simulink model "simThreeLinkFTC"  (R2014b)
settings: Solver=ode45  StartTime=0.0  StopTime=tof  FixedStep=dt  MaxStep=dtmax  RelTol=1e-3
values from neighbouring files (symbols this model uses):
  alpha = 1    [robotArmWith2Links.m]    (also in threeLinkFTC.m; twoLinkFTC.m; twoLinkFTCwAdaptive.m)
  Ar = [0 5; -30 -30]    [robotArmWith2Links.m]    (also in threeLinkFTC.m = [0 1; -5 -5]; twoLinkFTC.m = [0 10; -40 -40]; twoLinkFTCwAdaptive.m = [0 5; -250 -250])
  Arm1 = [0 1; -wn^2 -2*ksi*wn]    [robotArmWith2Links.m]    (also in threeLinkFTC.m; twoLinkFTC.m; twoLinkFTCwAdaptive.m)
  As = zeros(nofstates,nofstates)    [threeLinkFTC.m]    (also in twoLinkFDIbasisComparison.m; twoLinkFTC.m; twoLinkFTCwAdaptive.m)
  Brm1 = [0 wn^2]'    [robotArmWith2Links.m]    (also in threeLinkFTC.m; twoLinkFTC.m; twoLinkFTCwAdaptive.m)
  Dhat0 = zeros(6,1)    [threeLinkFTC.m]    (also in twoLinkFDIbasisComparison.m = zeros(4,1); twoLinkFTC.m = zeros(4,1); twoLinkFTCwAdaptive.m = zeros(4,1))
  Dlimit = 10    [threeLinkFTC.m]    (also in twoLinkFTC.m; twoLinkFTCwAdaptive.m)
  dtFc = 1*dtmax    (= 0.001)    [threeLinkFTC.m]    (also in twoLinkFDIbasisComparison.m; twoLinkFTC.m; twoLinkFTCwAdaptive.m)
  epsilon = 0.5    [robotArmWith2Links.m]    (also in threeLinkFTC.m; twoLinkFTC.m; twoLinkFTCwAdaptive.m)
  epsilontheta = 0.01    [threeLinkFTC.m]    (also in twoLinkFDIbasisComparison.m; twoLinkFTC.m; twoLinkFTCwAdaptive.m)
  faultyArm = 3    [threeLinkFTC.m]    (also in twoLinkFDIbasisComparison.m = 2; twoLinkFTC.m = 2; twoLinkFTCwAdaptive.m = 1)
  FDstart = 0.5    [threeLinkFTC.m]    (also in twoLinkFTC.m; twoLinkFTCwAdaptive.m)
  fmPosition = [0 90 -45]'*pi/180    [threeLinkFTC.m]    (also in twoLinkFTC.m = [90 0]'*pi/180; twoLinkFTCwAdaptive.m = [90 0]'*pi/180)
  g = 9.81    [robotArmWith2Links.m]    (also in threeLinkFTC.m; twoLinkFDIbasisComparison.m; twoLinkFTC.m; twoLinkFTCwAdaptive.m)
  GammaW = 1000    [threeLinkFTC.m]    (also in twoLinkFDIbasisComparison.m; twoLinkFTC.m; twoLinkFTCwAdaptive.m)
  I1 = 8.33e-2    (= 0.0833)    [robotArmWith2Links.m]    (also in threeLinkFTC.m = 0.0833333333333; twoLinkFDIbasisComparison.m = 0.0833333333333; twoLinkFTC.m = 0.0833333333333; twoLinkFTCwAdaptive.m = 0.0833333333333)
  I2 = 8.33e-2    (= 0.0833)    [robotArmWith2Links.m]    (also in threeLinkFTC.m = 0.0833333333333; twoLinkFDIbasisComparison.m = 0.0833333333333; twoLinkFTC.m = 0.0833333333333; twoLinkFTCwAdaptive.m = 0.0833333333333)
  I3 = m3*l3^2*1/12    (= 0.0833333333333)    [threeLinkFTC.m]
  ifault = 2    [threeLinkFTC.m]    (also in twoLinkFDIbasisComparison.m; twoLinkFTC.m; twoLinkFTCwAdaptive.m)
  K1 = 2*wn*ksi    (= 87.9645943005)    [robotArmWith2Links.m]    (also in threeLinkFTC.m = 8.79645943005; twoLinkFTC.m; twoLinkFTCwAdaptive.m = 43.9822971503)
  K2 = wn^2    (= 986.960440109)    [robotArmWith2Links.m]    (also in threeLinkFTC.m = 39.4784176044; twoLinkFTC.m; twoLinkFTCwAdaptive.m)
  Kp = wn^2    (= 157.913670417)    [threeLinkFTC.m]    (also in twoLinkFDIbasisComparison.m = 3947.84176044; twoLinkFTC.m = 3947.84176044; twoLinkFTCwAdaptive.m = 3947.84176044)
  Kv = 2*ksi*wn    (= 17.5929188601)    [threeLinkFTC.m]    (also in twoLinkFDIbasisComparison.m = 125.663706144; twoLinkFTC.m = 125.663706144; twoLinkFTCwAdaptive.m = 125.663706144)
  l1 = 1    [robotArmWith2Links.m]    (also in threeLinkFTC.m; twoLinkFDIbasisComparison.m; twoLinkFTC.m; twoLinkFTCwAdaptive.m)
  l2 = 1    [robotArmWith2Links.m]    (also in threeLinkFTC.m; twoLinkFDIbasisComparison.m; twoLinkFTC.m; twoLinkFTCwAdaptive.m)
  lc1 = l1/2    (= 0.5)    [robotArmWith2Links.m]    (also in threeLinkFTC.m; twoLinkFDIbasisComparison.m; twoLinkFTC.m; twoLinkFTCwAdaptive.m)
  lc2 = l2/2    (= 0.5)    [robotArmWith2Links.m]    (also in threeLinkFTC.m; twoLinkFDIbasisComparison.m; twoLinkFTC.m; twoLinkFTCwAdaptive.m)
  m1 = 1    [robotArmWith2Links.m]    (also in threeLinkFTC.m; twoLinkFDIbasisComparison.m; twoLinkFTC.m; twoLinkFTCwAdaptive.m)
  m2 = 1    [robotArmWith2Links.m]    (also in threeLinkFTC.m; twoLinkFDIbasisComparison.m; twoLinkFTC.m; twoLinkFTCwAdaptive.m)
  m3 = 1    [threeLinkFTC.m]
  nCheby = 4    [threeLinkFTC.m]    (also in twoLinkFDIbasisComparison.m; twoLinkFTC.m; twoLinkFTCwAdaptive.m)
  Ps = lyap(As(4:6,4:6)',Q)    [threeLinkFTC.m]    (also in twoLinkFDIbasisComparison.m = lyap(As(3:4,3:4)',Q); twoLinkFTC.m = lyap(As(3:4,3:4)',Q); twoLinkFTCwAdaptive.m = lyap(As(3:4,3:4)',Q))
  q0 = [80 20]'*pi/180    [robotArmWith2Links.m]    (also in threeLinkFTC.m = [90 0 0]'*pi/180; twoLinkFDIbasisComparison.m = [90 0]'*pi/180; twoLinkFTC.m = [90 0]'*pi/180; twoLinkFTCwAdaptive.m = [90 0]'*pi/180)
  qdot0 = [0 0]'    [robotArmWith2Links.m]    (also in threeLinkFTC.m = [0 0 0]'*pi/180; twoLinkFDIbasisComparison.m = [0 0]'*pi/180; twoLinkFTC.m = [0 0]'*pi/180; twoLinkFTCwAdaptive.m = [0 0]'*pi/180)
  r0 = [0 0]'    [robotArmWith2Links.m]    (also in threeLinkFTC.m; twoLinkFTC.m; twoLinkFTCwAdaptive.m)
  rmax = inf*[50*pi/180 inf]'    [robotArmWith2Links.m]    (also in threeLinkFTC.m; twoLinkFTC.m; twoLinkFTCwAdaptive.m)
  rmin = -rmax    [robotArmWith2Links.m]    (also in threeLinkFTC.m; twoLinkFTC.m; twoLinkFTCwAdaptive.m)
  tfault = 5    [threeLinkFTC.m]    (also in twoLinkFDIbasisComparison.m; twoLinkFTC.m; twoLinkFTCwAdaptive.m = 1)
  W0 = 0    [threeLinkFTC.m]    (also in twoLinkFDIbasisComparison.m; twoLinkFTC.m; twoLinkFTCwAdaptive.m)
  Wbnd = 1000    [threeLinkFTC.m]    (also in twoLinkFDIbasisComparison.m; twoLinkFTC.m; twoLinkFTCwAdaptive.m)
  xhat0 = [q0 ; qdot0]    [threeLinkFTC.m]    (also in twoLinkFDIbasisComparison.m; twoLinkFTC.m; twoLinkFTCwAdaptive.m)
undefined symbols (not defined in the file or in its folder): Intmax, Intmin
libraries: simulink x9, vrlib x3, dspbuff3 x1
(part 2 of 3)

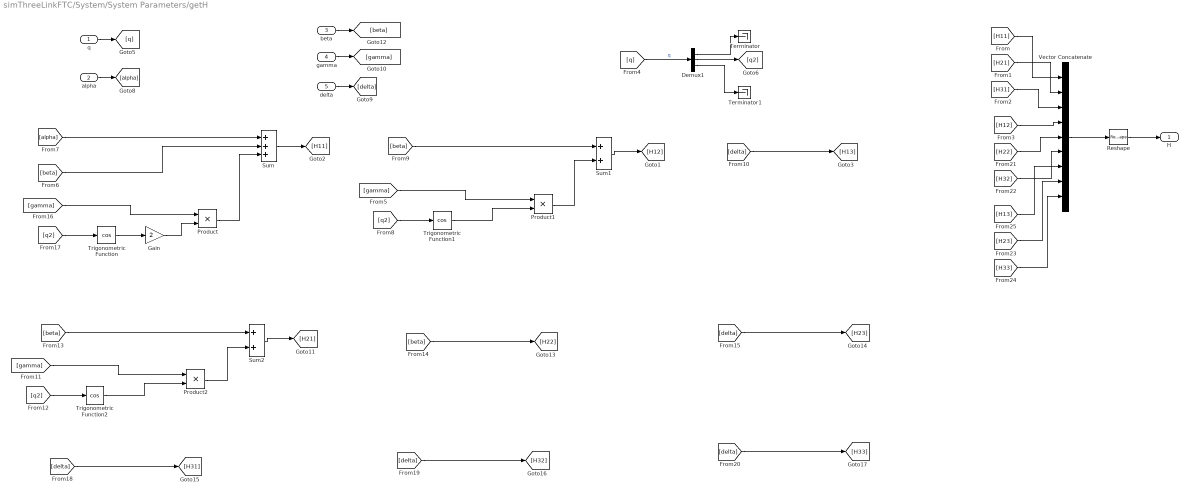
== system simThreeLinkFTC/System/System Parameters/getH ==
  q : Inport
  alpha : Inport  Port=2
  beta : Inport  Port=3
  gamma : Inport  Port=4
  delta : Inport  Port=5
  Demux1 : Demux  Outputs=3
  Gain : Gain  Gain=2
  Product : Product
  Product1 : Product
  Product2 : Product
  Reshape : Reshape  OutputDimensionality=Customize  OutputDimensions=[3,3]
  Sum : Sum  Inputs=+++
  Sum1 : Sum
  Sum2 : Sum
  Terminator : Terminator
  Terminator1 : Terminator
  Trigonometric Function : Trigonometry  Operator=cos
  Trigonometric Function1 : Trigonometry  Operator=cos
  Trigonometric Function2 : Trigonometry  Operator=cos
  Vector Concatenate : Concatenate  NumInputs=9
  H : Outport
  wires:
  Reshape/1 -> H/1
  Sum/1 -> [H11]
  q/1 -> [q]
  [q] -> Demux1/1  "q"
  Demux1/1 -> Terminator/1
  Demux1/3 -> Terminator1/1
  Demux1/2 -> [q2]
  alpha/1 -> [alpha]
  delta/1 -> [delta]
  gamma/1 -> [gamma]
  beta/1 -> [beta]
  [q2] -> Trigonometric Function/1
  Trigonometric Function/1 -> Gain/1
  [gamma] -> Product/1
  Gain/1 -> Product/2
  [alpha] -> Sum/1
  [beta] -> Sum/2
  Product/1 -> Sum/3
  Sum1/1 -> [H12]
  [q2] -> Trigonometric Function1/1
  [gamma] -> Product1/1
  Trigonometric Function1/1 -> Product1/2
  [beta] -> Sum1/1
  Product1/1 -> Sum1/2
  [delta] -> [H13]
  Sum2/1 -> [H21]
  [q2] -> Trigonometric Function2/1
  [gamma] -> Product2/1
  Trigonometric Function2/1 -> Product2/2
  [beta] -> Sum2/1
  Product2/1 -> Sum2/2
  [beta] -> [H22]
  [delta] -> [H23]
  [delta] -> [H31]
  [delta] -> [H32]
  [delta] -> [H33]
  Vector Concatenate/1 -> Reshape/1
  [H12] -> Vector Concatenate/4
  [H22] -> Vector Concatenate/5
  [H31] -> Vector Concatenate/3
  [H32] -> Vector Concatenate/6
  [H21] -> Vector Concatenate/2
  [H11] -> Vector Concatenate/1
  [H13] -> Vector Concatenate/7
  [H23] -> Vector Concatenate/8
  [H33] -> Vector Concatenate/9

== system simThreeLinkFTC/Controller/Disturbance Estimator/getDisturbance/Chebyshev Basis Functions ==
  x : Inport
  tau : Inport  Port=2
  Chebyshev Polynomail Value Calculation : Subsystem  TreatAsAtomicUnit=on
  Demux : Demux  Outputs=6
  Mux : Mux  Inputs=6
  Reshape1 : Reshape  OutputDimensionality=Column vector (2-D)
  Reshape2 : Reshape  OutputDimensionality=Column vector (2-D)
  Terminator1 : Terminator
  Tn : Outport
  wires:
  [Tn] -> Tn/1
  [z] -> Chebyshev Polynomail Value Calculation/1(x)
  Chebyshev Polynomail Value Calculation/1(chebyPol) -> Reshape2/1
  Reshape2/1 -> [Tn]
  tau/1 -> Terminator1/1
  x/1 -> [x]
  Mux/1 -> Reshape1/1
  Reshape1/1 -> [z]
  [x] -> Demux/1
  Demux/1 -> [q1]
  Demux/2 -> [q2]
  Demux/3 -> [q3]
  Demux/4 -> [q1dot]
  Demux/5 -> [q2dot]
  Demux/6 -> [q3dot]
  [q2] -> Mux/2
  [q3] -> Mux/3
  [q1] -> Mux/1
  [q1dot] -> Mux/4
  [q2dot] -> Mux/5
  [q3dot] -> Mux/6

== system simThreeLinkFTC/Controller/Disturbance Estimator/getDisturbance/getDhat ==
  psiz : Inport
  es : Inport  Port=2
  Bus Creator : BusCreator  Inputs=3
  Math Function : Math  Operator=transpose  SaturateOnIntegerOverflow=on
  Math Function1 : Math  Operator=transpose  SaturateOnIntegerOverflow=on
  Math Function2 : Math  Operator=transpose  SaturateOnIntegerOverflow=on
  Reshape : Reshape  OutputDimensionality=Column vector (2-D)
  Selector : Selector  NumberOfDimensions=2  InputPortWidth=3  IndexOptions=Select all,Index vector (dialog)  Indices=[1 3],1  OutputSizes=1,1
  Selector1 : Selector  NumberOfDimensions=2  InputPortWidth=3  IndexOptions=Select all,Index vector (dialog)  Indices=[1 3],2  OutputSizes=1,1
  Selector2 : Selector  NumberOfDimensions=2  InputPortWidth=3  IndexOptions=Select all,Index vector (dialog)  Indices=[1 3],3  OutputSizes=1,1
  Terminator1 : Terminator
  Vector Concatenate : Concatenate  NumInputs=3
  adaptiveGain : Subsystem  TreatAsAtomicUnit=on
  getW1 : Subsystem
  getW2 : Subsystem
  getW3 : Subsystem
  Dhat : Outport
  wires:
  es/1 -> [es]  "es"
  adaptiveGain/1(Wintegrand) -> [Wint]  "Wint"
  [Dhat] -> Dhat/1  "Dhat"
  psiz/1 -> [psiz]  "psiz"
  [es] -> adaptiveGain/2(es)
  [psiz] -> adaptiveGain/1(psi(z))
  [psiz] -> getW1/2(psiz)
  Selector/1 -> getW1/1(Wint)
  Vector Concatenate/1 -> Reshape/1
  [psiz] -> getW2/2(psiz)
  Selector1/1 -> getW2/1(Wint)
  Reshape/1 -> [Dhat]
  Bus Creator/1 -> Terminator1/1  "W"
  getW2/2(WTpsi) -> Vector Concatenate/2
  getW1/2(WTpsi) -> Vector Concatenate/1
  getW1/1(W) -> Math Function/1
  getW2/1(W) -> Math Function1/1
  [Wint] -> Selector2/1, Selector1/1, Selector/1
  Math Function/1 -> Bus Creator/1  "W1"
  Math Function1/1 -> Bus Creator/2  "W2"
  Selector2/1 -> getW3/1(Wint)
  [psiz] -> getW3/2(psiz)
  getW3/1(W) -> Math Function2/1
  Math Function2/1 -> Bus Creator/3
  getW3/2(WTpsi) -> Vector Concatenate/3  "W3"

== system simThreeLinkFTC/Controller/FTC Controller/1st Link Compensator/ ADI Controller ==
  qc : Inport
  q : Inport  Port=2
  qdot : Inport  Port=3
  Comp : Inport  Port=4
  1 : Selector  NumberOfDimensions=2  InputPortWidth=3  IndexOptions=Index vector (dialog),Index vector (dialog)  Indices=1,1  OutputSizes=1,1
  2 : Selector  NumberOfDimensions=2  InputPortWidth=3  IndexOptions=Index vector (dialog),Index vector (dialog)  Indices=1,1  OutputSizes=1,1
  3 : Selector  NumberOfDimensions=2  InputPortWidth=3  IndexOptions=Index vector (dialog),Index vector (dialog)  Indices=2,1  OutputSizes=1,1
  4 : Selector  NumberOfDimensions=2  InputPortWidth=3  IndexOptions=Index vector (dialog),Index vector (dialog)  Indices=2,1  OutputSizes=1,1
  Add : Sum  Inputs=+-+
  Add1 : Sum
  Add2 : Sum
  Constant2 : Constant  Value=2*pi
  Demux : Demux  Outputs=2
  Demux1 : Demux  Outputs=2
  Demux3 : Demux  Outputs=2
  Discrete-Time Integrator : DiscreteIntegrator  IntegratorMethod=Integration: Backward Euler  InitialCondition=r0  InitialConditionSetting=State (most efficient)  SampleTime=-1  LimitOutput=on  UpperSaturationLimit=rmax  LowerSaturationLimit=rmin
  Gain3 : Gain  Gain=[1/epsilon]'
  Gain4 : Gain  Gain=alpha
  Gain8 : Gain  Gain=Ar  Multiplication=Matrix(K*u)
  Math Function : Math  Operator=rem  SaturateOnIntegerOverflow=on
  Memory3 : Memory  X0=r0  InheritSampleTime=on  LinearizeMemory=on  LinearizeAsDelay=on
  Mux1 : Mux  Inputs=2
  Mux2 : Mux  Inputs=2
  Mux3 : Mux  Inputs=2
  Reference model : Subsystem  TreatAsAtomicUnit=on
  Reshape{1..4} (4 alike) : Reshape  OutputDimensionality=Column vector (2-D)
  System model : Subsystem  TreatAsAtomicUnit=on
  Terminator1 : Terminator
  Terminator3 : Terminator
  r : Outport
  wires:
  [Comp] -> Add/3
  Comp/1 -> [Comp]  "Comp"
  [r] -> 4/1
  Reshape4/1 -> r/1  "rp"
  Math Function/1 -> Mux3/2
  Mux3/1 -> Reshape4/1
  4/1 -> Mux3/1
  [r] -> Gain8/1
  1/1 -> Math Function/1
  [r] -> 3/1
  3/1 -> Mux2/2
  Demux1/2 -> Terminator3/1
  [qdot] -> Demux1/1
  Mux2/1 -> Reshape3/1
  Demux1/1 -> Mux2/1
  2/1 -> Add1/2
  [r] -> 2/1
  Demux/2 -> [r2]
  Demux/1 -> [r1]
  Reshape2/1 -> Memory3/1
  Discrete-Time Integrator/1 -> Reshape2/1
  Gain3/1 -> Discrete-Time Integrator/1
  [r] -> 1/1
  Constant2/1 -> Math Function/2
  Memory3/1 -> [r]  "r"
  Add1/1 -> Mux1/2
  [r2] -> Add1/1
  Demux3/2 -> Terminator1/1
  [q] -> Demux3/1
  Reshape1/1 -> System model/1(q)
  Mux1/1 -> Reshape1/1
  Demux3/1 -> Mux1/1
  Reshape3/1 -> System model/2(qdot)
  Gain8/1 -> Add2/2
  System model/1(f1) -> [f1]  "f1"
  Reference model/1(f1r) -> [f1r]  "f1r"
  [r1] -> Reference model/3(r1)  "r1"
  [q] -> Reference model/1(q)
  [qdot] -> Reference model/2(qdot)
  qdot/1 -> [qdot]
  q/1 -> [q]
  Add2/1 -> Gain3/1
  Gain4/1 -> Add2/1
  [f1r] -> Add/2
  [f1] -> Add/1
  Add/1 -> Gain4/1  "r_rhs"
  qc/1 -> Demux/1  "qc"

== system simThreeLinkFTC/Controller/FTC Controller/1st Link Compensator/Partial FBL q2 Controller ==
  qc : Inport
  qcdot : Inport  Port=2
  q : Inport  Port=3
  qdot : Inport  Port=4
  H : Inport  Port=5
  C : Inport  Port=6
  G : Inport  Port=7
  Collocated q2 Controller : Subsystem  TreatAsAtomicUnit=on
  Select 12_1 : Selector  NumberOfDimensions=2  InputPortWidth=3  IndexOptions=Index vector (dialog),Index vector (dialog)  Indices=[2 3],1  OutputSizes=1,1
  Select 12_2 : Selector  NumberOfDimensions=2  InputPortWidth=3  IndexOptions=Index vector (dialog),Index vector (dialog)  Indices=[2 3],1  OutputSizes=1,1
  Torque calculation : Subsystem  TreatAsAtomicUnit=on
  tau : Outport
  v : Outport  Port=2
  wires:
  [qdot] -> Torque calculation/5(qdot)
  Select 12_2/1 -> Collocated q2 Controller/4(qdot)
  [qdot] -> Select 12_2/1
  Select 12_1/1 -> Collocated q2 Controller/3(q)
  qc/1 -> [qc]
  qcdot/1 -> [qcdot]
  [tau] -> tau/1
  [qcdot] -> Collocated q2 Controller/2(rdot)
  [v] -> v/1
  qdot/1 -> [qdot]
  q/1 -> [q]
  [qc] -> Collocated q2 Controller/1(r)
  [G] -> Torque calculation/4(G)
  [C] -> Torque calculation/3(C)
  [H] -> Torque calculation/2(H)
  [v] -> Torque calculation/1(v)
  Torque calculation/1(tau) -> [tau]
  G/1 -> [G]
  H/1 -> [H]
  C/1 -> [C]
  Collocated q2 Controller/1(v) -> [v]  "v"
  [q] -> Select 12_1/1

== system simThreeLinkFTC/Controller/FTC Controller/3rd Link Compensator/ ADI Controller ==
  qc : Inport
  q : Inport  Port=2
  qdot : Inport  Port=3
  Comp : Inport  Port=4
  1 : Selector  NumberOfDimensions=2  InputPortWidth=3  IndexOptions=Index vector (dialog),Index vector (dialog)  Indices=1,1  OutputSizes=1,1
  3 : Selector  InputPortWidth=2  Indices=2
  4 : Selector  NumberOfDimensions=2  InputPortWidth=3  IndexOptions=Index vector (dialog),Index vector (dialog)  Indices=2,1  OutputSizes=1,1
  5 : Selector  InputPortWidth=2
  Add : Sum  Inputs=+-+
  Add1 : Sum
  Add2 : Sum
  Constant2 : Constant  Value=2*pi
  Discrete-Time Integrator : DiscreteIntegrator  IntegratorMethod=Integration: Backward Euler  InitialCondition=r0  InitialConditionSetting=State (most efficient)  SampleTime=-1  LimitOutput=on  UpperSaturationLimit=rmax  LowerSaturationLimit=rmin
  Gain3 : Gain  Gain=[1/epsilon]'
  Gain4 : Gain  Gain=alpha
  Gain8 : Gain  Gain=Ar  Multiplication=Matrix(K*u)
  Math Function : Math  Operator=rem  SaturateOnIntegerOverflow=on
  Memory3 : Memory  X0=r0  InheritSampleTime=on  LinearizeMemory=on  LinearizeAsDelay=on
  Mux1 : Mux  Inputs=3
  Mux2 : Mux  Inputs=3
  Mux3 : Mux  Inputs=2
  Reference model : Subsystem  TreatAsAtomicUnit=on
  Reshape{1..4} (4 alike) : Reshape  OutputDimensionality=Column vector (2-D)
  Selec t 1 : Selector  InputPortWidth=3
  Selec t 2 : Selector  InputPortWidth=3
  Selec t 3 : Selector  NumberOfDimensions=2  InputPortWidth=3  IndexOptions=Index vector (dialog),Index vector (dialog)  Indices=3,1  OutputSizes=1,1
  Selec t 4 : Selector  InputPortWidth=3  Indices=3
  Selec t 5 : Selector  InputPortWidth=3  Indices=3
  Selec t 6 : Selector  NumberOfDimensions=2  InputPortWidth=3  IndexOptions=Index vector (dialog),Index vector (dialog)  Indices=[1 2],1  OutputSizes=1,1
  System model : Subsystem  TreatAsAtomicUnit=on
  r : Outport
  wires:
  Add/1 -> Gain4/1  "r_rhs"
  [f1] -> Add/1
  [f1r] -> Add/2
  Gain4/1 -> Add2/1
  Add2/1 -> Gain3/1
  q/1 -> [q]
  qdot/1 -> [qdot]
  [qdot] -> Reference model/2(qdot)
  [q] -> Reference model/1(q)
  [r1] -> Reference model/3(r1)  "r1"
  Reference model/1(f1r) -> [f1r]  "f1r"
  System model/1(f1) -> [f1]  "f1"
  Gain8/1 -> Add2/2
  Reshape3/1 -> System model/2(qdot)
  Mux1/1 -> Reshape1/1
  Reshape1/1 -> System model/1(q)
  [r2] -> Add1/1
  Add1/1 -> Mux1/2
  Memory3/1 -> [r]  "r"
  Constant2/1 -> Math Function/2
  [r] -> 1/1
  Gain3/1 -> Discrete-Time Integrator/1
  Discrete-Time Integrator/1 -> Reshape2/1
  Reshape2/1 -> Memory3/1
  [r] -> 5/1
  5/1 -> Add1/2
  Mux2/1 -> Reshape3/1
  3/1 -> Mux2/2
  [r] -> 3/1
  1/1 -> Math Function/1
  [r] -> Gain8/1
  Mux3/1 -> Reshape4/1
  Reshape4/1 -> r/1  "rp"
  [r] -> 4/1
  Comp/1 -> [Comp]  "Comp"
  [Comp] -> Add/3
  qc/1 -> Selec t 3/1, Selec t 6/1  "qc"
  Selec t 3/1 -> [r1]
  [q] -> Selec t 1/1
  Selec t 1/1 -> Mux1/1
  [qdot] -> Selec t 2/1
  Selec t 2/1 -> Mux2/1
  [q] -> Selec t 4/1
  Selec t 4/1 -> Mux1/3
  [qdot] -> Selec t 5/1
  Selec t 5/1 -> Mux2/3
  Selec t 6/1 -> [r2]
  Math Function/1 -> Mux3/1
  4/1 -> Mux3/2

== system simThreeLinkFTC/Controller/FTC Controller/3rd Link Compensator/Partial FBL q2 Controller ==
  qc : Inport
  qcdot : Inport  Port=2
  q : Inport  Port=3
  qdot : Inport  Port=4
  H : Inport  Port=5
  C : Inport  Port=6
  G : Inport  Port=7
  Collocated q2 Controller : Subsystem  TreatAsAtomicUnit=on
  Select 12_1 : Selector  NumberOfDimensions=2  InputPortWidth=3  IndexOptions=Index vector (dialog),Index vector (dialog)  Indices=[1 2],1  OutputSizes=1,1
  Select 12_2 : Selector  NumberOfDimensions=2  InputPortWidth=3  IndexOptions=Index vector (dialog),Index vector (dialog)  Indices=[1 2],1  OutputSizes=1,1
  Torque calculation : Subsystem  TreatAsAtomicUnit=on
  tau : Outport
  v : Outport  Port=2
  wires:
  [q] -> Select 12_1/1
  Collocated q2 Controller/1(v) -> [v]  "v"
  C/1 -> [C]
  H/1 -> [H]
  G/1 -> [G]
  Torque calculation/1(tau) -> [tau]
  [v] -> Torque calculation/1(v)
  [H] -> Torque calculation/2(H)
  [C] -> Torque calculation/3(C)
  [G] -> Torque calculation/4(G)
  [qc] -> Collocated q2 Controller/1(r)
  q/1 -> [q]
  qdot/1 -> [qdot]
  [v] -> v/1
  [qcdot] -> Collocated q2 Controller/2(rdot)
  [tau] -> tau/1
  qcdot/1 -> [qcdot]
  qc/1 -> [qc]
  Select 12_1/1 -> Collocated q2 Controller/3(q)
  [qdot] -> Select 12_2/1
  Select 12_2/1 -> Collocated q2 Controller/4(qdot)
  [qdot] -> Torque calculation/5(qdot)

== system simThreeLinkFTC/Controller/Disturbance Estimator/getDisturbance/Chebyshev Basis Functions/Chebyshev Polynomail Value Calculation ==
  x : Inport
  Delay Line : dspbuff3/Delay Line  siz=nCheby  ic=zeros(nCheby,1)  directfeed=on  enable_output=off  hold_output=off  TreatMby1Signals=M channels (this choice will be removed - see release notes)
  For Iterator : ForIterator  IterationLimit=nCheby
  Frame Conversion : FrameConversion  OutFrame=Sample-based
  If : If  IfExpression=u1 > 2
  If Action Subsystem : Subsystem  TreatAsAtomicUnit=on
  If Action Subsystem1 : Subsystem  TreatAsAtomicUnit=on
  Memory : Memory  InheritSampleTime=on  LinearizeMemory=on  LinearizeAsDelay=on
  Merge : Merge
  Reshape : Reshape  OutputDimensionality=Column vector (2-D)
  chebyPol : Outport
  wires:
  For Iterator/1 -> [N]
  x/1 -> [x]
  [N] -> If/1
  If/1 -> If Action Subsystem/Action
  If/2 -> If Action Subsystem1/Action
  [N] -> If Action Subsystem1/2(N)
  [x] -> If Action Subsystem1/1(x)
  [x] -> If Action Subsystem/1(x)
  If Action Subsystem/1(polyval) -> Merge/1
  If Action Subsystem1/1(polval) -> Merge/2
  Merge/1 -> [polyval]
  [polyval] -> Delay Line/1
  Delay Line/1 -> Frame Conversion/1
  Reshape/1 -> [polyvals]
  [polyvals] -> Memory/1
  [polyvals] -> chebyPol/1  "chebyPol"
  Frame Conversion/1 -> Reshape/1
  Memory/1 -> If Action Subsystem/2(polyvals)

== system simThreeLinkFTC/Controller/Disturbance Estimator/getDisturbance/getDhat/adaptiveGain ==
  psi(z) : Inport
  es : Inport  Port=2
  Gain1 : Gain  Gain=-1
  Math Function : Math  Operator=transpose  SaturateOnIntegerOverflow=on
  P : Constant  Value=Ps  VectorParams1D=off
  Product1 : Product  Multiplication=Matrix(*)  RndMeth=Zero
  Product3 : Product  Multiplication=Matrix(*)  RndMeth=Zero
  Wintegrand : Outport
  wires:
  Product1/1 -> Product3/2
  psi(z)/1 -> Product3/1
  Gain1/1 -> Wintegrand/1
  es/1 -> Math Function/1
  Math Function/1 -> Product1/1
  P/1 -> Product1/2
  Product3/1 -> Gain1/1

== system simThreeLinkFTC/Controller/Disturbance Estimator/getDisturbance/getDhat/getW1 ==
  Wint : Inport
  psiz : Inport  Port=2
  Constant : Constant  Value=Wbnd  VectorParams1D=off
  Constant1 : Constant  Value=epsilontheta
  Discrete-Time Integrator : DiscreteIntegrator  IntegratorMethod=Integration: Trapezoidal  InitialCondition=W0  SampleTime=-1  LimitOutput=on  UpperSaturationLimit=Wbnd  LowerSaturationLimit=-Wbnd
  Gain : Gain  Gain=GammaW
  Math Function : Math  Operator=transpose  SaturateOnIntegerOverflow=on
  Memory4 : Memory  X0=W0  InheritSampleTime=on  LinearizeMemory=on  LinearizeAsDelay=on
  Product : Product  Multiplication=Matrix(*)  RndMeth=Zero
  Projection : Subsystem  TreatAsAtomicUnit=on
  W : Outport
  WTpsi : Outport  Port=2
  wires:
  [WTpsi] -> WTpsi/1
  [Wint] -> Projection/2(y)
  Math Function/1 -> Product/1
  [psiz] -> Product/2
  Discrete-Time Integrator/1 -> Math Function/1, [W], Memory4/1
  Gain/1 -> Discrete-Time Integrator/1
  Projection/1(Proj) -> Gain/1  "WintProj"
  Memory4/1 -> Projection/1(theta)
  Constant/1 -> Projection/3(Thetamax)
  Constant1/1 -> Projection/4(epsilontheta)
  [W] -> W/1
  Wint/1 -> [Wint]
  psiz/1 -> [psiz]
  Product/1 -> [WTpsi]  "WTpsi"

== system simThreeLinkFTC/Controller/Disturbance Estimator/getDisturbance/getDhat/getW2 ==
  Wint : Inport
  psiz : Inport  Port=2
  Constant : Constant  Value=Wbnd  VectorParams1D=off
  Constant1 : Constant  Value=epsilontheta
  Discrete-Time Integrator : DiscreteIntegrator  IntegratorMethod=Integration: Trapezoidal  InitialCondition=W0  SampleTime=-1  LimitOutput=on  UpperSaturationLimit=Wbnd  LowerSaturationLimit=-Wbnd
  Gain : Gain  Gain=GammaW
  Math Function : Math  Operator=transpose  SaturateOnIntegerOverflow=on
  Memory4 : Memory  X0=W0  InheritSampleTime=on  LinearizeMemory=on  LinearizeAsDelay=on
  Product : Product  Multiplication=Matrix(*)  RndMeth=Zero
  Projection : Subsystem  TreatAsAtomicUnit=on
  W : Outport
  WTpsi : Outport  Port=2
  wires:
  Product/1 -> [WTpsi]  "WTpsi"
  psiz/1 -> [psiz]
  Wint/1 -> [Wint]
  [W] -> W/1
  Constant1/1 -> Projection/4(epsilontheta)
  Constant/1 -> Projection/3(Thetamax)
  Memory4/1 -> Projection/1(theta)
  Projection/1(Proj) -> Gain/1  "WintProj"
  Gain/1 -> Discrete-Time Integrator/1
  Discrete-Time Integrator/1 -> Memory4/1, [W], Math Function/1
  [psiz] -> Product/2
  Math Function/1 -> Product/1
  [Wint] -> Projection/2(y)
  [WTpsi] -> WTpsi/1

== system simThreeLinkFTC/Controller/Disturbance Estimator/getDisturbance/getDhat/getW3 ==
  Wint : Inport
  psiz : Inport  Port=2
  Constant : Constant  Value=Wbnd  VectorParams1D=off
  Constant1 : Constant  Value=epsilontheta
  Discrete-Time Integrator : DiscreteIntegrator  IntegratorMethod=Integration: Trapezoidal  InitialCondition=W0  SampleTime=-1  LimitOutput=on  UpperSaturationLimit=Wbnd  LowerSaturationLimit=-Wbnd
  Gain : Gain  Gain=GammaW
  Math Function : Math  Operator=transpose  SaturateOnIntegerOverflow=on
  Memory4 : Memory  X0=W0  InheritSampleTime=on  LinearizeMemory=on  LinearizeAsDelay=on
  Product : Product  Multiplication=Matrix(*)  RndMeth=Zero
  Projection : Subsystem  TreatAsAtomicUnit=on
  W : Outport
  WTpsi : Outport  Port=2
  wires:
  [WTpsi] -> WTpsi/1
  [Wint] -> Projection/2(y)
  Math Function/1 -> Product/1
  [psiz] -> Product/2
  Discrete-Time Integrator/1 -> Math Function/1, [W], Memory4/1
  Gain/1 -> Discrete-Time Integrator/1
  Projection/1(Proj) -> Gain/1  "WintProj"
  Memory4/1 -> Projection/1(theta)
  Constant/1 -> Projection/3(Thetamax)
  Constant1/1 -> Projection/4(epsilontheta)
  [W] -> W/1
  Wint/1 -> [Wint]
  psiz/1 -> [psiz]
  Product/1 -> [WTpsi]  "WTpsi"

== system simThreeLinkFTC/Controller/FTC Controller/1st Link Compensator/ ADI Controller/Reference model ==
  q : Inport
  qdot : Inport  Port=2
  r1 : Inport  Port=3
  Add : Sum
  Constant : Constant  Value=Arm1  VectorParams1D=off
  Constant1 : Constant  Value=Brm1  VectorParams1D=off
  Demux2 : Demux  Outputs=2
  Demux3 : Demux  Outputs=2
  Mux : Mux  Inputs=2
  Product1 : Product  Multiplication=Matrix(*)
  Product3 : Product  Multiplication=Matrix(*)
  Reshape : Reshape  OutputDimensionality=Column vector (2-D)
  Terminator4 : Terminator
  Terminator5 : Terminator
  f1r : Outport
  wires:
  Add/1 -> [f1r]
  Product1/1 -> Add/2
  Product3/1 -> Add/1
  [r1] -> Product1/2
  Constant1/1 -> Product1/1
  Reshape/1 -> Product3/2
  Mux/1 -> Reshape/1
  [q1] -> Mux/1
  [q1dot] -> Mux/2
  [q2] -> Terminator5/1
  [q2dot] -> Terminator4/1
  [f1r] -> f1r/1
  Constant/1 -> Product3/1
  r1/1 -> [r1]
  Demux2/1 -> [q1]
  Demux2/2 -> [q2]
  Demux3/1 -> [q1dot]
  Demux3/2 -> [q2dot]
  q/1 -> Demux2/1
  qdot/1 -> Demux3/1

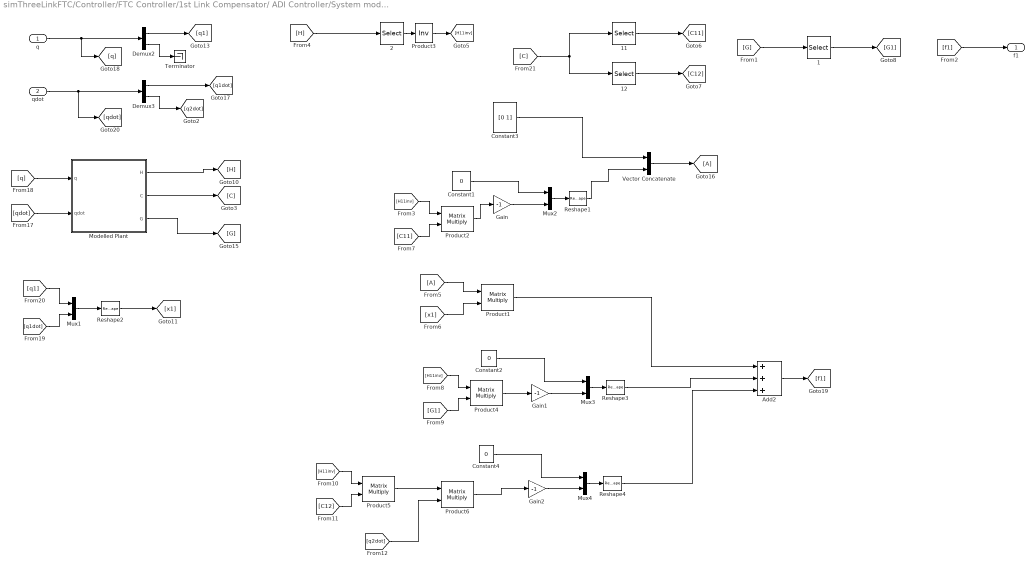
== system simThreeLinkFTC/Controller/FTC Controller/1st Link Compensator/ ADI Controller/System model ==
  q : Inport
  qdot : Inport  Port=2
  1 : Selector  NumberOfDimensions=2  InputPortWidth=3  IndexOptions=Index vector (dialog),Index vector (dialog)  Indices=1,1  OutputSizes=1,1
  11 : Selector  NumberOfDimensions=2  InputPortWidth=3  IndexOptions=Index vector (dialog),Index vector (dialog)  Indices=1,1  OutputSizes=1,1
  12 : Selector  NumberOfDimensions=2  InputPortWidth=3  IndexOptions=Index vector (dialog),Index vector (dialog)  Indices=1,2  OutputSizes=1,1
  2 : Selector  NumberOfDimensions=2  InputPortWidth=3  IndexOptions=Index vector (dialog),Index vector (dialog)  Indices=1,1  OutputSizes=1,1
  Add2 : Sum  Inputs=+++
  Constant1 : Constant  Value=0  VectorParams1D=off
  Constant2 : Constant  Value=0  VectorParams1D=off
  Constant3 : Constant  Value=[0 1]  VectorParams1D=off
  Constant4 : Constant  Value=0  VectorParams1D=off
  Demux2 : Demux  Outputs=2
  Demux3 : Demux  Outputs=2
  Gain : Gain  Gain=-1
  Gain1 : Gain  Gain=-1
  Gain2 : Gain  Gain=-1
  Modelled Plant : Subsystem  TreatAsAtomicUnit=on
  Mux{1..4} (4 alike) : Mux  Inputs=2
  Product{1..2,4..6} (5 alike) : Product  Multiplication=Matrix(*)  RndMeth=Zero
  Product3 : Product  Inputs=/  Multiplication=Matrix(*)  RndMeth=Zero
  Reshape1 : Reshape  OutputDimensionality=Row vector (2-D)
  Reshape2 : Reshape  OutputDimensionality=Column vector (2-D)
  Reshape3 : Reshape  OutputDimensionality=Column vector (2-D)
  Reshape4 : Reshape  OutputDimensionality=Column vector (2-D)
  Terminator : Terminator
  Vector Concatenate : Concatenate  Mode=Multidimensional array
  f1 : Outport
  wires:
  Reshape4/1 -> Add2/3
  Reshape3/1 -> Add2/2
  Product6/1 -> Gain2/1
  [q2dot] -> Product6/2
  Product5/1 -> Product6/1
  Gain2/1 -> Mux4/2
  Mux4/1 -> Reshape4/1
  Constant4/1 -> Mux4/1
  [C12] -> Product5/2
  [H11inv] -> Product5/1
  Gain1/1 -> Mux3/2
  Mux3/1 -> Reshape3/1
  Constant2/1 -> Mux3/1
  Product4/1 -> Gain1/1
  Gain/1 -> Mux2/2
  [G1] -> Product4/2
  [H11inv] -> Product4/1
  [x1] -> Product1/2
  [A] -> Product1/1
  Vector Concatenate/1 -> [A]
  Reshape1/1 -> Vector Concatenate/2
  Constant3/1 -> Vector Concatenate/1
  Mux2/1 -> Reshape1/1
  Constant1/1 -> Mux2/1
  Product2/1 -> Gain/1
  Reshape2/1 -> [x1]
  Mux1/1 -> Reshape2/1
  [q1] -> Mux1/1
  [q1dot] -> Mux1/2
  [q] -> Modelled Plant/1(q)
  [qdot] -> Modelled Plant/2(qdot)
  Modelled Plant/3(G) -> [G]
  Modelled Plant/2(C) -> [C]
  Modelled Plant/1(H) -> [H]
  [C11] -> Product2/2
  [H11inv] -> Product2/1
  Add2/1 -> [f1]
  Product1/1 -> Add2/1
  Product3/1 -> [H11inv]
  2/1 -> Product3/1
  [H] -> 2/1
  Demux2/1 -> [q1]
  Demux2/2 -> Terminator/1
  Demux3/1 -> [q1dot]
  Demux3/2 -> [q2dot]
  q/1 -> Demux2/1, [q]
  qdot/1 -> Demux3/1, [qdot]
  1/1 -> [G1]
  [G] -> 1/1
  12/1 -> [C12]
  11/1 -> [C11]
  [C] -> 11/1, 12/1
  [f1] -> f1/1

== system simThreeLinkFTC/Controller/FTC Controller/1st Link Compensator/Partial FBL q2 Controller/Collocated q2 Controller ==
  r : Inport
  rdot : Inport  Port=2
  q : Inport  Port=3
  qdot : Inport  Port=4
  Add3 : Sum
  Gain2 : Gain  Gain=-K1
  Gain3 : Gain  Gain=-K2
  sum1 : Sum  Inputs=+-
  sum2 : Sum  Inputs=+-
  v : Outport
  wires:
  rdot/1 -> [rdot]  "rdot"
  sum2/1 -> [edot]  "edot"
  [rdot] -> sum2/2
  [qdot] -> sum2/1
  [v] -> v/1  "v"
  r/1 -> [r]  "r"
  sum1/1 -> [e]  "e"
  [r] -> sum1/2
  [q] -> sum1/1
  q/1 -> [q]  "q"
  qdot/1 -> [qdot]  "qdot"
  [edot] -> Gain2/1
  [e] -> Gain3/1
  Gain2/1 -> Add3/1
  Gain3/1 -> Add3/2
  Add3/1 -> [v]

== system simThreeLinkFTC/Controller/FTC Controller/1st Link Compensator/Partial FBL q2 Controller/Torque calculation ==
  v : Inport
  H : Inport  Port=2
  C : Inport  Port=3
  G : Inport  Port=4
  qdot : Inport  Port=5
  1 : Selector  NumberOfDimensions=2  InputPortWidth=3  IndexOptions=Index vector (dialog),Index vector (dialog)  Indices=[1],1  OutputSizes=1,1
  11 : Selector  NumberOfDimensions=2  InputPortWidth=3  IndexOptions=Index vector (dialog),Index vector (dialog)  Indices=1,1  OutputSizes=1,1
  12-13 : Selector  NumberOfDimensions=2  InputPortWidth=3  IndexOptions=Index vector (dialog),Index vector (dialog)  Indices=1,[2 3]  OutputSizes=1,1
  2-3 : Selector  NumberOfDimensions=2  InputPortWidth=3  IndexOptions=Index vector (dialog),Index vector (dialog)  Indices=[2 3],1  OutputSizes=1,1
  21-31 : Selector  NumberOfDimensions=2  InputPortWidth=3  IndexOptions=Index vector (dialog),Index vector (dialog)  Indices=[2 3],1  OutputSizes=1,1
  22-33 : Selector  NumberOfDimensions=2  InputPortWidth=3  IndexOptions=Index vector (dialog),Index vector (dialog)  Indices=[2 3],[2 3]  OutputSizes=1,1
  Product : Product  Inputs=/  Multiplication=Matrix(*)  RndMeth=Zero
  Product{1..4,6..7} (6 alike) : Product  Multiplication=Matrix(*)  RndMeth=Zero
  Product5 : Product  Inputs=/  Multiplication=Matrix(*)  RndMeth=Zero
  Sum of Elements1 : Sum  Inputs=+-+
  Sum of Elements2 : Sum
  Sum of Elements3 : Sum  Inputs=+-
  tau : Outport
  wires:
  [qdotp] -> [qdot]
  qdot/1 -> [qdotp]
  2-3/1 -> [Phi2]
  1/1 -> [Phi1]
  22-33/1 -> [H22]
  21-31/1 -> [H21]
  12-13/1 -> [H12]
  11/1 -> [H11]
  Sum of Elements2/1 -> 2-3/1, 1/1
  [G] -> Sum of Elements2/2
  Product2/1 -> Sum of Elements2/1
  [qdot] -> Product2/2
  [C] -> Product2/1
  [Hp] -> 22-33/1, 21-31/1, 12-13/1, 11/1
  G/1 -> [Gp]
  H/1 -> [Hp]
  C/1 -> [Cp]
  Product3/1 -> Sum of Elements1/3
  Product4/1 -> Sum of Elements1/2
  [Phi2] -> Sum of Elements1/1
  [Phi1] -> Product4/2
  Sum of Elements3/1 -> [Hbar]
  Product7/1 -> Sum of Elements3/2
  [H22] -> Sum of Elements3/1
  [H12] -> Product7/2
  Product6/1 -> Product7/1
  Product5/1 -> Product6/2
  [H21] -> Product6/1
  [H11] -> Product5/1
  Sum of Elements1/1 -> [tau]
  [v] -> Product3/2
  [Hbar] -> Product3/1
  Product1/1 -> Product4/1
  Product/1 -> Product1/2
  [H21] -> Product1/1
  [H11] -> Product/1
  v/1 -> [v]
  [tau] -> tau/1
  [Gp] -> [G]
  [Cp] -> [C]

== system simThreeLinkFTC/Controller/FTC Controller/3rd Link Compensator/ ADI Controller/Reference model ==
  q : Inport
  qdot : Inport  Port=2
  r1 : Inport  Port=3
  Add : Sum
  Constant : Constant  Value=Arm1  VectorParams1D=off
  Constant1 : Constant  Value=Brm1  VectorParams1D=off
  Mux : Mux  Inputs=2
  Product1 : Product  Multiplication=Matrix(*)
  Product3 : Product  Multiplication=Matrix(*)
  Reshape : Reshape  OutputDimensionality=Column vector (2-D)
  Selec t 1 : Selector  NumberOfDimensions=2  InputPortWidth=3  IndexOptions=Index vector (dialog),Index vector (dialog)  Indices=3,1  OutputSizes=1,1
  Selec t 3 : Selector  NumberOfDimensions=2  InputPortWidth=3  IndexOptions=Index vector (dialog),Index vector (dialog)  Indices=3,1  OutputSizes=1,1
  f1r : Outport
  wires:
  q/1 -> Selec t 3/1
  r1/1 -> [r1]
  Constant/1 -> Product3/1
  [f1r] -> f1r/1
  [q1dot] -> Mux/2
  [q1] -> Mux/1
  Mux/1 -> Reshape/1
  Reshape/1 -> Product3/2
  Constant1/1 -> Product1/1
  [r1] -> Product1/2
  Product3/1 -> Add/1
  Product1/1 -> Add/2
  Add/1 -> [f1r]
  Selec t 3/1 -> [q1]
  qdot/1 -> Selec t 1/1
  Selec t 1/1 -> [q1dot]

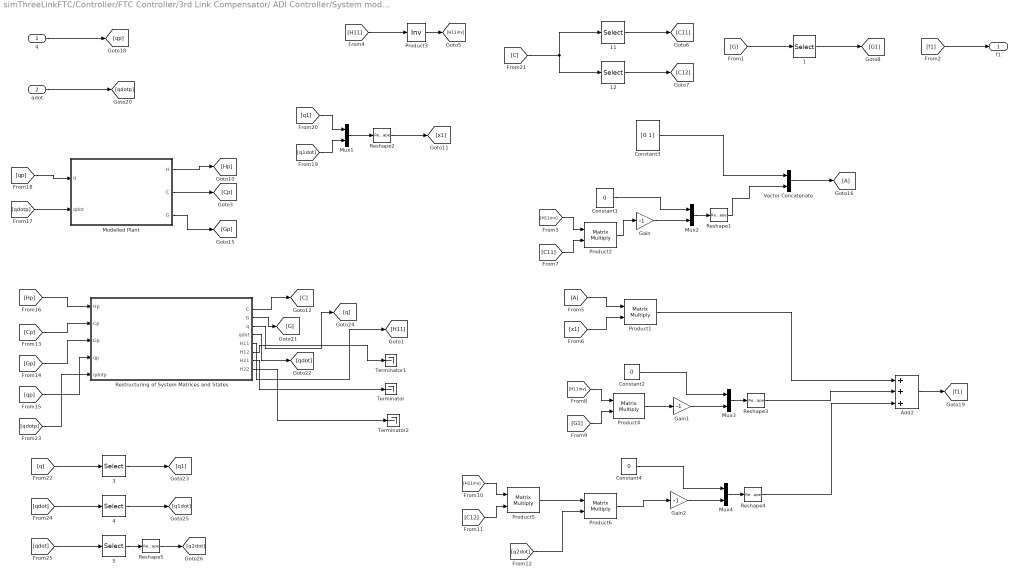
== system simThreeLinkFTC/Controller/FTC Controller/3rd Link Compensator/ ADI Controller/System model ==
  q : Inport
  qdot : Inport  Port=2
  1 : Selector  NumberOfDimensions=2  InputPortWidth=3  IndexOptions=Index vector (dialog),Index vector (dialog)  Indices=1,1  OutputSizes=1,1
  11 : Selector  NumberOfDimensions=2  InputPortWidth=3  IndexOptions=Index vector (dialog),Index vector (dialog)  Indices=1,1  OutputSizes=1,1
  12 : Selector  NumberOfDimensions=2  InputPortWidth=3  IndexOptions=Index vector (dialog),Index vector (dialog)  Indices=1,[2 3]  OutputSizes=1,1
  3 : Selector  InputPortWidth=3
  4 : Selector  InputPortWidth=3
  5 : Selector  InputPortWidth=3  Indices=[2 3]
  Add2 : Sum  Inputs=+++
  Constant1 : Constant  Value=0  VectorParams1D=off
  Constant2 : Constant  Value=0  VectorParams1D=off
  Constant3 : Constant  Value=[0 1]  VectorParams1D=off
  Constant4 : Constant  Value=0  VectorParams1D=off
  Gain : Gain  Gain=-1
  Gain1 : Gain  Gain=-1
  Gain2 : Gain  Gain=-1
  Modelled Plant : Subsystem
  Mux{1..4} (4 alike) : Mux  Inputs=2
  Product{1..2,4..6} (5 alike) : Product  Multiplication=Matrix(*)  RndMeth=Zero
  Product3 : Product  Inputs=/  Multiplication=Matrix(*)  RndMeth=Zero
  Reshape1 : Reshape  OutputDimensionality=Row vector (2-D)
  Reshape{2..5} (4 alike) : Reshape  OutputDimensionality=Column vector (2-D)
  Restructuring of System Matrices and States : Subsystem
  Terminator : Terminator
  Terminator1 : Terminator
  Terminator2 : Terminator
  Vector Concatenate : Concatenate  Mode=Multidimensional array
  f1 : Outport
  wires:
  [f1] -> f1/1
  [C] -> 12/1, 11/1
  11/1 -> [C11]
  12/1 -> [C12]
  [G] -> 1/1
  1/1 -> [G1]
  qdot/1 -> [qdotp]
  [H11] -> Product3/1
  Product3/1 -> [H11inv]
  Product1/1 -> Add2/1
  Add2/1 -> [f1]
  [H11inv] -> Product2/1
  [C11] -> Product2/2
  Modelled Plant/1(H) -> [Hp]
  Modelled Plant/2(C) -> [Cp]
  Modelled Plant/3(G) -> [Gp]
  [qdotp] -> Modelled Plant/2(qdot)
  [q1dot] -> Mux1/2
  [q1] -> Mux1/1
  Mux1/1 -> Reshape2/1
  Reshape2/1 -> [x1]
  Product2/1 -> Gain/1
  Constant1/1 -> Mux2/1
  Mux2/1 -> Reshape1/1
  Constant3/1 -> Vector Concatenate/1
  Reshape1/1 -> Vector Concatenate/2
  Vector Concatenate/1 -> [A]
  [A] -> Product1/1
  [x1] -> Product1/2
  [H11inv] -> Product4/1
  [G1] -> Product4/2
  Gain/1 -> Mux2/2
  Product4/1 -> Gain1/1
  Constant2/1 -> Mux3/1
  Mux3/1 -> Reshape3/1
  Gain1/1 -> Mux3/2
  [H11inv] -> Product5/1
  [C12] -> Product5/2
  Constant4/1 -> Mux4/1
  Mux4/1 -> Reshape4/1
  Gain2/1 -> Mux4/2
  Product5/1 -> Product6/1
  [q2dot] -> Product6/2
  Product6/1 -> Gain2/1
  Reshape3/1 -> Add2/2
  Reshape4/1 -> Add2/3
  [Hp] -> Restructuring of System Matrices and States/1(Hp)
  [Cp] -> Restructuring of System Matrices and States/2(Cp)
  [Gp] -> Restructuring of System Matrices and States/3(Gp)
  [qp] -> Restructuring of System Matrices and States/4(qp)
  Restructuring of System Matrices and States/1(C) -> [C]
  Restructuring of System Matrices and States/2(G) -> [G]
  Restructuring of System Matrices and States/4(qdot) -> [qdot]
  Restructuring of System Matrices and States/5(H11) -> [H11]
  Restructuring of System Matrices and States/6(H12) -> Terminator1/1
  Restructuring of System Matrices and States/7(H21) -> Terminator/1
  Restructuring of System Matrices and States/8(H22) -> Terminator2/1
  [q] -> 3/1
  3/1 -> [q1]
  Restructuring of System Matrices and States/3(q) -> [q]
  [qdotp] -> Restructuring of System Matrices and States/5(qdotp)
  [qdot] -> 4/1
  4/1 -> [q1dot]
  [qdot] -> 5/1
  Reshape5/1 -> [q2dot]
  5/1 -> Reshape5/1
  q/1 -> [qp]
  [qp] -> Modelled Plant/1(q)

== system simThreeLinkFTC/Controller/FTC Controller/3rd Link Compensator/Partial FBL q2 Controller/Collocated q2 Controller ==
  r : Inport
  rdot : Inport  Port=2
  q : Inport  Port=3
  qdot : Inport  Port=4
  Add3 : Sum
  Gain2 : Gain  Gain=-K1
  Gain3 : Gain  Gain=-K2
  sum1 : Sum  Inputs=+-
  sum2 : Sum  Inputs=+-
  v : Outport
  wires:
  Add3/1 -> [v]
  Gain3/1 -> Add3/2
  Gain2/1 -> Add3/1
  [e] -> Gain3/1
  [edot] -> Gain2/1
  qdot/1 -> [qdot]  "qdot"
  q/1 -> [q]  "q"
  [q] -> sum1/1
  [r] -> sum1/2
  sum1/1 -> [e]  "e"
  r/1 -> [r]  "r"
  [v] -> v/1  "v"
  [qdot] -> sum2/1
  [rdot] -> sum2/2
  sum2/1 -> [edot]  "edot"
  rdot/1 -> [rdot]  "rdot"

== system simThreeLinkFTC/Controller/FTC Controller/3rd Link Compensator/Partial FBL q2 Controller/Torque calculation ==
  v : Inport
  H : Inport  Port=2
  C : Inport  Port=3
  G : Inport  Port=4
  qdot : Inport  Port=5
  1 : Selector  NumberOfDimensions=2  InputPortWidth=3  IndexOptions=Index vector (dialog),Index vector (dialog)  Indices=[1],1  OutputSizes=1,1
  2-3 : Selector  NumberOfDimensions=2  InputPortWidth=3  IndexOptions=Index vector (dialog),Index vector (dialog)  Indices=[2 3],1  OutputSizes=1,1
  Product : Product  Inputs=/  Multiplication=Matrix(*)  RndMeth=Zero
  Product{1..4,6..7} (6 alike) : Product  Multiplication=Matrix(*)  RndMeth=Zero
  Product5 : Product  Inputs=/  Multiplication=Matrix(*)  RndMeth=Zero
  Restructuring of System Matrices and States : Subsystem
  Sum of Elements1 : Sum  Inputs=+-+
  Sum of Elements2 : Sum
  Sum of Elements3 : Sum  Inputs=+-
  tau : Outport
  wires:
  [tau] -> tau/1
  v/1 -> [v]
  [H11] -> Product/1
  [H21] -> Product1/1
  Product/1 -> Product1/2
  Product1/1 -> Product4/1
  [Hbar] -> Product3/1
  [v] -> Product3/2
  Sum of Elements1/1 -> [tau]
  [H11] -> Product5/1
  [H21] -> Product6/1
  Product5/1 -> Product6/2
  Product6/1 -> Product7/1
  [H12] -> Product7/2
  [H22] -> Sum of Elements3/1
  Product7/1 -> Sum of Elements3/2
  Sum of Elements3/1 -> [Hbar]
  [Phi1] -> Product4/2
  [Phi2] -> Sum of Elements1/1
  Product4/1 -> Sum of Elements1/2
  Product3/1 -> Sum of Elements1/3
  C/1 -> [Cp]
  H/1 -> [Hp]
  G/1 -> [Gp]
  [C] -> Product2/1
  [qdot] -> Product2/2
  Product2/1 -> Sum of Elements2/1
  [G] -> Sum of Elements2/2
  Sum of Elements2/1 -> 1/1, 2-3/1
  1/1 -> [Phi1]
  2-3/1 -> [Phi2]
  qdot/1 -> [qdotp]
  [Hp] -> Restructuring of System Matrices and States/1(Hp)
  [Cp] -> Restructuring of System Matrices and States/2(Cp)
  [Gp] -> Restructuring of System Matrices and States/3(Gp)
  [qdotp] -> Restructuring of System Matrices and States/4(qdotp)
  Restructuring of System Matrices and States/1(C) -> [C]
  Restructuring of System Matrices and States/2(G) -> [G]
  Restructuring of System Matrices and States/3(qdot) -> [qdot]
  Restructuring of System Matrices and States/4(H11) -> [H11]
  Restructuring of System Matrices and States/5(H12) -> [H12]
  Restructuring of System Matrices and States/6(H21) -> [H21]
  Restructuring of System Matrices and States/7(H22) -> [H22]

== system simThreeLinkFTC/Controller/Disturbance Estimator/getDisturbance/Chebyshev Basis Functions/Chebyshev Polynomail Value Calculation/If Action Subsystem ==
  x : Inport
  polyvals : Inport  Port=2
  Action Port : ActionPort  PropagateVarSize=During execution  ActionType=then
  Add : Sum  Inputs=+-
  Constant : Constant  Value=nCheby
  Constant1 : Constant  Value=nCheby-1
  Gain : Gain  Gain=2
  Product : Product  RndMeth=Zero
  Selector : Selector  IndexOptions=Index vector (port)  Indices=[1 3]
  Selector1 : Selector  IndexOptions=Index vector (port)  Indices=[1 3]
  polyval : Outport
  wires:
  x/1 -> [x]
  polyvals/1 -> [polyvals]  "if.polyvals"
  [polyvals] -> Selector/1
  Constant1/1 -> Selector/2
  Selector/1 -> [Tm2]  "Tm2"
  [polyvals] -> Selector1/1
  Constant/1 -> Selector1/2
  Selector1/1 -> [Tm1]  "Tm1"
  [x] -> Product/1
  [Tm1] -> Product/2
  Product/1 -> Gain/1
  Gain/1 -> Add/1
  [Tm2] -> Add/2
  Add/1 -> polyval/1  "if.polyval"

== system simThreeLinkFTC/Controller/Disturbance Estimator/getDisturbance/Chebyshev Basis Functions/Chebyshev Polynomail Value Calculation/If Action Subsystem1 ==
  x : Inport
  N : Inport  Port=2
  Action Port : ActionPort  PropagateVarSize=During execution  ActionType=else
  Bias1 : Bias  Bias=-1
  Data Type Conversion : DataTypeConversion
  Math Function : Math  Operator=pow  OutputSignalType=real  SaturateOnIntegerOverflow=on
  polval : Outport
  wires:
  x/1 -> Math Function/1
  N/1 -> Bias1/1  "else.N"
  Math Function/1 -> polval/1  "else.polyval"
  Data Type Conversion/1 -> Math Function/2
  Bias1/1 -> Data Type Conversion/1

== system simThreeLinkFTC/Controller/Disturbance Estimator/getDisturbance/getDhat/getW1/Projection ==
  theta : Inport
  y : Inport  Port=2
  Thetamax : Inport  Port=3
  epsilontheta : Inport  Port=4
  Bias : Bias  Bias=1
  Bias1 : Bias  Bias=1
  Divide : Product  Inputs=*/
  Divide1 : Product  Inputs=*/
  Dot Product : DotProduct  InputSameDT=on  OutDataTypeStr=Inherit: Inherit via internal rule
  Gain : Gain  Gain=2
  Math Function : Math  Operator=square  SaturateOnIntegerOverflow=on
  Math Function1 : Math  Operator=square  SaturateOnIntegerOverflow=on
  Normalize Vector1 : vrlib/Utilities/Normalize Vector  maxzero=0
  Product{,1..3,6..7} (6 alike) : Product  RndMeth=Zero
  Product4 : Product  Multiplication=Matrix(*)  RndMeth=Zero
  Product5 : Product  Multiplication=Matrix(*)  RndMeth=Zero
  Reshape : Reshape  OutputDimensionality=Row vector (2-D)
  Reshape1 : Reshape  OutputDimensionality=Row vector (2-D)
  Sum4 : Sum  Inputs=|+-
  Sum5 : Sum  Inputs=|+-
  Switch : Switch  Criteria=u2 > Threshold
  Switch1 : Switch  Criteria=u2 > Threshold
  Proj : Outport
  wires:
  [f] -> Switch/2
  y/1 -> [y]
  Switch/1 -> Proj/1
  Product5/1 -> Switch1/2
  [y] -> Product5/2
  Sum4/1 -> Divide/1
  Math Function/1 -> Sum4/2, Product2/1
  Product4/1 -> Product3/2
  [theta] -> Reshape1/1, Product4/2
  [df] -> Reshape/1
  Reshape/1 -> Product5/1
  Reshape1/1 -> Product4/1
  theta/1 -> [theta]
  [y] -> Switch/3
  Switch1/1 -> Switch/1
  [y] -> Sum5/1
  Product/1 -> Product1/1
  [y] -> Switch1/3
  Product1/1 -> Sum5/2
  Sum5/1 -> Switch1/1
  [f] -> Product1/2
  [df] -> Normalize Vector1/1
  Normalize Vector1/1 -> Dot Product/1, Product/1
  [y] -> Dot Product/2
  Dot Product/1 -> Product/2
  Thetamax/1 -> [Thetamax]
  [Thetamax] -> Math Function/1
  epsilontheta/1 -> [epsilontheta]
  [epsilontheta] -> Product2/2
  Product2/1 -> Divide/2
  Divide/1 -> [f]
  Product3/1 -> Sum4/1
  Bias/1 -> Product3/1
  [epsilontheta] -> Bias/1
  [epsilontheta] -> Bias1/1, Product6/1
  Bias1/1 -> Gain/1
  Gain/1 -> Divide1/1
  [Thetamax] -> Math Function1/1
  Math Function1/1 -> Product6/2
  Product6/1 -> Divide1/2
  Product7/1 -> [df]
  [theta] -> Product7/1
  Divide1/1 -> Product7/2

== system simThreeLinkFTC/Controller/Disturbance Estimator/getDisturbance/getDhat/getW2/Projection ==
  theta : Inport
  y : Inport  Port=2
  Thetamax : Inport  Port=3
  epsilontheta : Inport  Port=4
  Bias : Bias  Bias=1
  Bias1 : Bias  Bias=1
  Divide : Product  Inputs=*/
  Divide1 : Product  Inputs=*/
  Dot Product : DotProduct  InputSameDT=on  OutDataTypeStr=Inherit: Inherit via internal rule
  Gain : Gain  Gain=2
  Math Function : Math  Operator=square  SaturateOnIntegerOverflow=on
  Math Function1 : Math  Operator=square  SaturateOnIntegerOverflow=on
  Normalize Vector1 : vrlib/Utilities/Normalize Vector  maxzero=0
  Product{,1..3,6..7} (6 alike) : Product  RndMeth=Zero
  Product4 : Product  Multiplication=Matrix(*)  RndMeth=Zero
  Product5 : Product  Multiplication=Matrix(*)  RndMeth=Zero
  Reshape : Reshape  OutputDimensionality=Row vector (2-D)
  Reshape1 : Reshape  OutputDimensionality=Row vector (2-D)
  Sum4 : Sum  Inputs=|+-
  Sum5 : Sum  Inputs=|+-
  Switch : Switch  Criteria=u2 > Threshold
  Switch1 : Switch  Criteria=u2 > Threshold
  Proj : Outport
  wires:
  Divide1/1 -> Product7/2
  [theta] -> Product7/1
  Product7/1 -> [df]
  Product6/1 -> Divide1/2
  Math Function1/1 -> Product6/2
  [Thetamax] -> Math Function1/1
  Gain/1 -> Divide1/1
  Bias1/1 -> Gain/1
  [epsilontheta] -> Product6/1, Bias1/1
  [epsilontheta] -> Bias/1
  Bias/1 -> Product3/1
  Product3/1 -> Sum4/1
  Divide/1 -> [f]
  Product2/1 -> Divide/2
  [epsilontheta] -> Product2/2
  epsilontheta/1 -> [epsilontheta]
  [Thetamax] -> Math Function/1
  Thetamax/1 -> [Thetamax]
  Dot Product/1 -> Product/2
  [y] -> Dot Product/2
  Normalize Vector1/1 -> Product/1, Dot Product/1
  [df] -> Normalize Vector1/1
  [f] -> Product1/2
  Sum5/1 -> Switch1/1
  Product1/1 -> Sum5/2
  [y] -> Switch1/3
  Product/1 -> Product1/1
  [y] -> Sum5/1
  Switch1/1 -> Switch/1
  [y] -> Switch/3
  theta/1 -> [theta]
  Reshape1/1 -> Product4/1
  Reshape/1 -> Product5/1
  [df] -> Reshape/1
  [theta] -> Product4/2, Reshape1/1
  Product4/1 -> Product3/2
  Math Function/1 -> Product2/1, Sum4/2
  Sum4/1 -> Divide/1
  [y] -> Product5/2
  Product5/1 -> Switch1/2
  Switch/1 -> Proj/1
  y/1 -> [y]
  [f] -> Switch/2

== system simThreeLinkFTC/Controller/Disturbance Estimator/getDisturbance/getDhat/getW3/Projection ==
  theta : Inport
  y : Inport  Port=2
  Thetamax : Inport  Port=3
  epsilontheta : Inport  Port=4
  Bias : Bias  Bias=1
  Bias1 : Bias  Bias=1
  Divide : Product  Inputs=*/
  Divide1 : Product  Inputs=*/
  Dot Product : DotProduct  InputSameDT=on  OutDataTypeStr=Inherit: Inherit via internal rule
  Gain : Gain  Gain=2
  Math Function : Math  Operator=square  SaturateOnIntegerOverflow=on
  Math Function1 : Math  Operator=square  SaturateOnIntegerOverflow=on
  Normalize Vector1 : vrlib/Utilities/Normalize Vector  maxzero=0
  Product{,1..3,6..7} (6 alike) : Product  RndMeth=Zero
  Product4 : Product  Multiplication=Matrix(*)  RndMeth=Zero
  Product5 : Product  Multiplication=Matrix(*)  RndMeth=Zero
  Reshape : Reshape  OutputDimensionality=Row vector (2-D)
  Reshape1 : Reshape  OutputDimensionality=Row vector (2-D)
  Sum4 : Sum  Inputs=|+-
  Sum5 : Sum  Inputs=|+-
  Switch : Switch  Criteria=u2 > Threshold
  Switch1 : Switch  Criteria=u2 > Threshold
  Proj : Outport
  wires:
  [f] -> Switch/2
  y/1 -> [y]
  Switch/1 -> Proj/1
  Product5/1 -> Switch1/2
  [y] -> Product5/2
  Sum4/1 -> Divide/1
  Math Function/1 -> Sum4/2, Product2/1
  Product4/1 -> Product3/2
  [theta] -> Reshape1/1, Product4/2
  [df] -> Reshape/1
  Reshape/1 -> Product5/1
  Reshape1/1 -> Product4/1
  theta/1 -> [theta]
  [y] -> Switch/3
  Switch1/1 -> Switch/1
  [y] -> Sum5/1
  Product/1 -> Product1/1
  [y] -> Switch1/3
  Product1/1 -> Sum5/2
  Sum5/1 -> Switch1/1
  [f] -> Product1/2
  [df] -> Normalize Vector1/1
  Normalize Vector1/1 -> Dot Product/1, Product/1
  [y] -> Dot Product/2
  Dot Product/1 -> Product/2
  Thetamax/1 -> [Thetamax]
  [Thetamax] -> Math Function/1
  epsilontheta/1 -> [epsilontheta]
  [epsilontheta] -> Product2/2
  Product2/1 -> Divide/2
  Divide/1 -> [f]
  Product3/1 -> Sum4/1
  Bias/1 -> Product3/1
  [epsilontheta] -> Bias/1
  [epsilontheta] -> Bias1/1, Product6/1
  Bias1/1 -> Gain/1
  Gain/1 -> Divide1/1
  [Thetamax] -> Math Function1/1
  Math Function1/1 -> Product6/2
  Product6/1 -> Divide1/2
  Product7/1 -> [df]
  [theta] -> Product7/1
  Divide1/1 -> Product7/2

== system simThreeLinkFTC/Controller/FTC Controller/1st Link Compensator/ ADI Controller/System model/Modelled Plant ==
  q : Inport
  qdot : Inport  Port=2
  Demux : Demux  Outputs=2
  Demux1 : Demux  Outputs=2
  Demux2 : Demux  Outputs=2
  Sum of Elements : Sum  Inputs=+
  Terminator4 : Terminator
  Terminator5 : Terminator
  Terminator6 : Terminator
  Trigonometric Function : Trigonometry
  Trigonometric Function1 : Trigonometry  Operator=cos
  Trigonometric Function2 : Trigonometry
  Trigonometric Function3 : Trigonometry  Operator=cos
  get Plant Parameters : Subsystem
  getC : Subsystem
  getG : Subsystem
  getH : Subsystem
  H : Outport
  C : Outport  Port=2
  G : Outport  Port=3
  wires:
  [qdot] -> get Plant Parameters/4(qdot)
  [G] -> get Plant Parameters/3(G)
  [H] -> get Plant Parameters/1(H)
  [C] -> get Plant Parameters/2(C)
  get Plant Parameters/1(busData) -> Terminator6/1  "ModeledSystem"
  [G] -> G/1
  [C] -> C/1
  [H] -> H/1
  Trigonometric Function3/1 -> [c12]
  Demux2/2 -> [q2dot]
  Demux2/1 -> [q1dot]
  qdot/1 -> [qdot], Demux2/1
  Trigonometric Function2/1 -> Terminator5/1
  Sum of Elements/1 -> Trigonometric Function3/1, Trigonometric Function2/1
  Trigonometric Function1/1 -> Demux1/1
  Demux1/2 -> [c2]
  Demux1/1 -> [c1]
  Demux/2 -> [s2]
  Demux/1 -> Terminator4/1
  Trigonometric Function/1 -> Demux/1
  q/1 -> Sum of Elements/1, Trigonometric Function1/1, Trigonometric Function/1
  getG/1(G) -> [G]
  [c12] -> getG/2(c12)
  [c1] -> getG/1(c1)
  getC/1(C) -> [C]
  getH/1(H) -> [H]
  [q2dot] -> getC/3(q2dot)
  [q1dot] -> getC/2(q1dot)
  [s2] -> getC/1(s2)
  [c2] -> getH/1(c2)

== system simThreeLinkFTC/Controller/FTC Controller/3rd Link Compensator/ ADI Controller/System model/Modelled Plant ==
  q : Inport
  qdot : Inport  Port=2
  Constant : Constant  Value=I1+m1*lc1^2+m2*l1^2+m3*l1^2  VectorParams1D=off
  Constant2 : Constant  Value=[0 0 0]'  VectorParams1D=off
  Constant3 : Constant  Value=I2+I3+m2*lc2^2+m3*l2^2  VectorParams1D=off
  Constant4 : Constant  Value=m2*l1*lc2+m3*l1*l2  VectorParams1D=off
  Constant5 : Constant  Value=I3  VectorParams1D=off
  getC : Subsystem
  getH : Subsystem
  H : Outport
  C : Outport  Port=2
  G : Outport  Port=3
  wires:
  q/1 -> [q]
  qdot/1 -> [qdot]
  getH/1(H) -> [H]
  Constant2/1 -> [G]
  [H] -> H/1
  Constant/1 -> [alpha]
  [G] -> G/1
  [C] -> C/1
  Constant3/1 -> [beta]
  Constant4/1 -> [gamma]
  Constant5/1 -> [delta]
  [alpha] -> getH/2(alpha)
  [beta] -> getH/3(beta)
  [gamma] -> getH/4(gamma)
  [delta] -> getH/5(delta)
  [q] -> getH/1(q)
  getC/1(C) -> [C]
  [alpha] -> getC/3(alpha)
  [beta] -> getC/4(beta)
  [gamma] -> getC/5(gamma)
  [delta] -> getC/6(delta)
  [q] -> getC/1(q)
  [qdot] -> getC/2(qdot)
